simulink model "c960x4096_x14_7_r2013b_frb"  (R2013b)
settings: Solver=ode45  StartTime=0.0  StopTime=40960  RelTol=1e-3
undefined symbols (not defined in the file): sfp
libraries: xbsIndex_r4 x14620, casper_library_misc x61, dspsigops x32, casper_library_multipliers x24, simulink x18, xps_library x18
(part 9 of 79)

== system c960x4096_x14_7_r2013b_frb/cross_corr/cross_multiplier ==
  sync_in : Inport
  din0 : Inport  Port=2
  din1 : Inport  Port=3
  c_to_ri0_{0..7} (8 alike) : casper_library_misc/c_to_ri  n_bits=bit_width_in  bin_pt=binary_point_in
  c_to_ri1_{0..7} (8 alike) : casper_library_misc/c_to_ri  n_bits=bit_width_in  bin_pt=binary_point_in
  cmult0_0_{0..7} (8 alike) : casper_library_multipliers/cmult_4bit_hdl*  mult_latency=mult_latency  add_latency=add_latency
  cmult0_1_{0..7} (8 alike) : casper_library_multipliers/cmult_4bit_hdl*  mult_latency=mult_latency  add_latency=add_latency
  cmult1_0_{0..7} (8 alike) : casper_library_multipliers/cmult_4bit_hdl*  mult_latency=mult_latency  add_latency=add_latency
  cvrt0_0_0_imag : Subsystem  AncestorBlock=casper_library_misc/convert_of  mask(convert_of){bit_width_i=37, binary_point_i=34, bit_width_o=37, binary_point_o=34, latency=0, overflow=Wrap, quantization=Truncate}
      mask prompts: bit_width_i "Bit Width In"; binary_point_i "Binary Point In"; bit_width_o "Bit Width Out"; binary_point_o "Binary Point Out"; overflow "Overflow Behaviour"; quantization "Quantization Behaviour"
      mask help:
      | Converts from one 2's complement bit-width
      | and/or binary point position to another.
      | Includes underflow/overflow indicator.
      mask init:
      | convert_of_init(gcb, ...
      |     'bit_width_i', bit_width_i, ...
      |     'binary_point_i', binary_point_i, ...
      |     'bit_width_o', bit_width_o, ...
      |     'binary_point_o', binary_point_o, ...
      |     'latency', latency, ...
      |     'overflow', overflow, ...
      |     'quantization', quantization);
      settings: AttributesFormatString=[37,34]->[37,34]
      mask TypeOptions overflow: Wrap | Saturate | Error
      mask TypeOptions quantization: Truncate | Round  (unbiased: +/- Inf) | Round  (unbiased: even values)
  cvrt0_0_0_real : Subsystem  AncestorBlock=casper_library_misc/convert_of  mask(convert_of){bit_width_i=37, binary_point_i=34, bit_width_o=37, binary_point_o=34, latency=0, overflow=Wrap, quantization=Truncate}
      mask prompts: bit_width_i "Bit Width In"; binary_point_i "Binary Point In"; bit_width_o "Bit Width Out"; binary_point_o "Binary Point Out"; overflow "Overflow Behaviour"; quantization "Quantization Behaviour"
      mask help:
      | Converts from one 2's complement bit-width
      | and/or binary point position to another.
      | Includes underflow/overflow indicator.
      mask init: same as c960x4096_x14_7_r2013b_frb/cross_corr/cross_multiplier/cvrt0_0_0_imag
      settings: AttributesFormatString=[37,34]->[37,34]
      mask TypeOptions overflow: Wrap | Saturate | Error
      mask TypeOptions quantization: Truncate | Round  (unbiased: +/- Inf) | Round  (unbiased: even values)
  cvrt0_0_1_imag : Subsystem  AncestorBlock=casper_library_misc/convert_of  mask(convert_of){bit_width_i=37, binary_point_i=34, bit_width_o=37, binary_point_o=34, latency=0, overflow=Wrap, quantization=Truncate}
      mask prompts: bit_width_i "Bit Width In"; binary_point_i "Binary Point In"; bit_width_o "Bit Width Out"; binary_point_o "Binary Point Out"; overflow "Overflow Behaviour"; quantization "Quantization Behaviour"
      mask help:
      | Converts from one 2's complement bit-width
      | and/or binary point position to another.
      | Includes underflow/overflow indicator.
      mask init: same as c960x4096_x14_7_r2013b_frb/cross_corr/cross_multiplier/cvrt0_0_0_imag
      settings: AttributesFormatString=[37,34]->[37,34]
      mask TypeOptions overflow: Wrap | Saturate | Error
      mask TypeOptions quantization: Truncate | Round  (unbiased: +/- Inf) | Round  (unbiased: even values)
  cvrt0_0_1_real : Subsystem  AncestorBlock=casper_library_misc/convert_of  mask(convert_of){bit_width_i=37, binary_point_i=34, bit_width_o=37, binary_point_o=34, latency=0, overflow=Wrap, quantization=Truncate}
      mask prompts: bit_width_i "Bit Width In"; binary_point_i "Binary Point In"; bit_width_o "Bit Width Out"; binary_point_o "Binary Point Out"; overflow "Overflow Behaviour"; quantization "Quantization Behaviour"
      mask help:
      | Converts from one 2's complement bit-width
      | and/or binary point position to another.
      | Includes underflow/overflow indicator.
      mask init: same as c960x4096_x14_7_r2013b_frb/cross_corr/cross_multiplier/cvrt0_0_0_imag
      settings: AttributesFormatString=[37,34]->[37,34]
      mask TypeOptions overflow: Wrap | Saturate | Error
      mask TypeOptions quantization: Truncate | Round  (unbiased: +/- Inf) | Round  (unbiased: even values)
  cvrt0_0_2_imag : Subsystem  AncestorBlock=casper_library_misc/convert_of  mask(convert_of){bit_width_i=37, binary_point_i=34, bit_width_o=37, binary_point_o=34, latency=0, overflow=Wrap, quantization=Truncate}
      mask prompts: bit_width_i "Bit Width In"; binary_point_i "Binary Point In"; bit_width_o "Bit Width Out"; binary_point_o "Binary Point Out"; overflow "Overflow Behaviour"; quantization "Quantization Behaviour"
      mask help:
      | Converts from one 2's complement bit-width
      | and/or binary point position to another.
      | Includes underflow/overflow indicator.
      mask init: same as c960x4096_x14_7_r2013b_frb/cross_corr/cross_multiplier/cvrt0_0_0_imag
      settings: AttributesFormatString=[37,34]->[37,34]
      mask TypeOptions overflow: Wrap | Saturate | Error
      mask TypeOptions quantization: Truncate | Round  (unbiased: +/- Inf) | Round  (unbiased: even values)
  cvrt0_0_2_real : Subsystem  AncestorBlock=casper_library_misc/convert_of  mask(convert_of){bit_width_i=37, binary_point_i=34, bit_width_o=37, binary_point_o=34, latency=0, overflow=Wrap, quantization=Truncate}
      mask prompts: bit_width_i "Bit Width In"; binary_point_i "Binary Point In"; bit_width_o "Bit Width Out"; binary_point_o "Binary Point Out"; overflow "Overflow Behaviour"; quantization "Quantization Behaviour"
      mask help:
      | Converts from one 2's complement bit-width
      | and/or binary point position to another.
      | Includes underflow/overflow indicator.
      mask init: same as c960x4096_x14_7_r2013b_frb/cross_corr/cross_multiplier/cvrt0_0_0_imag
      settings: AttributesFormatString=[37,34]->[37,34]
      mask TypeOptions overflow: Wrap | Saturate | Error
      mask TypeOptions quantization: Truncate | Round  (unbiased: +/- Inf) | Round  (unbiased: even values)
  cvrt0_0_3_imag : Subsystem  AncestorBlock=casper_library_misc/convert_of  mask(convert_of){bit_width_i=37, binary_point_i=34, bit_width_o=37, binary_point_o=34, latency=0, overflow=Wrap, quantization=Truncate}
      mask prompts: bit_width_i "Bit Width In"; binary_point_i "Binary Point In"; bit_width_o "Bit Width Out"; binary_point_o "Binary Point Out"; overflow "Overflow Behaviour"; quantization "Quantization Behaviour"
      mask help:
      | Converts from one 2's complement bit-width
      | and/or binary point position to another.
      | Includes underflow/overflow indicator.
      mask init: same as c960x4096_x14_7_r2013b_frb/cross_corr/cross_multiplier/cvrt0_0_0_imag
      settings: AttributesFormatString=[37,34]->[37,34]
      mask TypeOptions overflow: Wrap | Saturate | Error
      mask TypeOptions quantization: Truncate | Round  (unbiased: +/- Inf) | Round  (unbiased: even values)
  cvrt0_0_3_real : Subsystem  AncestorBlock=casper_library_misc/convert_of  mask(convert_of){bit_width_i=37, binary_point_i=34, bit_width_o=37, binary_point_o=34, latency=0, overflow=Wrap, quantization=Truncate}
      mask prompts: bit_width_i "Bit Width In"; binary_point_i "Binary Point In"; bit_width_o "Bit Width Out"; binary_point_o "Binary Point Out"; overflow "Overflow Behaviour"; quantization "Quantization Behaviour"
      mask help:
      | Converts from one 2's complement bit-width
      | and/or binary point position to another.
      | Includes underflow/overflow indicator.
      mask init: same as c960x4096_x14_7_r2013b_frb/cross_corr/cross_multiplier/cvrt0_0_0_imag
      settings: AttributesFormatString=[37,34]->[37,34]
      mask TypeOptions overflow: Wrap | Saturate | Error
      mask TypeOptions quantization: Truncate | Round  (unbiased: +/- Inf) | Round  (unbiased: even values)
  cvrt0_0_4_imag : Subsystem  AncestorBlock=casper_library_misc/convert_of  mask(convert_of){bit_width_i=37, binary_point_i=34, bit_width_o=37, binary_point_o=34, latency=0, overflow=Wrap, quantization=Truncate}
      mask prompts: bit_width_i "Bit Width In"; binary_point_i "Binary Point In"; bit_width_o "Bit Width Out"; binary_point_o "Binary Point Out"; overflow "Overflow Behaviour"; quantization "Quantization Behaviour"
      mask help:
      | Converts from one 2's complement bit-width
      | and/or binary point position to another.
      | Includes underflow/overflow indicator.
      mask init: same as c960x4096_x14_7_r2013b_frb/cross_corr/cross_multiplier/cvrt0_0_0_imag
      settings: AttributesFormatString=[37,34]->[37,34]
      mask TypeOptions overflow: Wrap | Saturate | Error
      mask TypeOptions quantization: Truncate | Round  (unbiased: +/- Inf) | Round  (unbiased: even values)
  cvrt0_0_4_real : Subsystem  AncestorBlock=casper_library_misc/convert_of  mask(convert_of){bit_width_i=37, binary_point_i=34, bit_width_o=37, binary_point_o=34, latency=0, overflow=Wrap, quantization=Truncate}
      mask prompts: bit_width_i "Bit Width In"; binary_point_i "Binary Point In"; bit_width_o "Bit Width Out"; binary_point_o "Binary Point Out"; overflow "Overflow Behaviour"; quantization "Quantization Behaviour"
      mask help:
      | Converts from one 2's complement bit-width
      | and/or binary point position to another.
      | Includes underflow/overflow indicator.
      mask init: same as c960x4096_x14_7_r2013b_frb/cross_corr/cross_multiplier/cvrt0_0_0_imag
      settings: AttributesFormatString=[37,34]->[37,34]
      mask TypeOptions overflow: Wrap | Saturate | Error
      mask TypeOptions quantization: Truncate | Round  (unbiased: +/- Inf) | Round  (unbiased: even values)
  cvrt0_0_5_imag : Subsystem  AncestorBlock=casper_library_misc/convert_of  mask(convert_of){bit_width_i=37, binary_point_i=34, bit_width_o=37, binary_point_o=34, latency=0, overflow=Wrap, quantization=Truncate}
      mask prompts: bit_width_i "Bit Width In"; binary_point_i "Binary Point In"; bit_width_o "Bit Width Out"; binary_point_o "Binary Point Out"; overflow "Overflow Behaviour"; quantization "Quantization Behaviour"
      mask help:
      | Converts from one 2's complement bit-width
      | and/or binary point position to another.
      | Includes underflow/overflow indicator.
      mask init: same as c960x4096_x14_7_r2013b_frb/cross_corr/cross_multiplier/cvrt0_0_0_imag
      settings: AttributesFormatString=[37,34]->[37,34]
      mask TypeOptions overflow: Wrap | Saturate | Error
      mask TypeOptions quantization: Truncate | Round  (unbiased: +/- Inf) | Round  (unbiased: even values)
  cvrt0_0_5_real : Subsystem  AncestorBlock=casper_library_misc/convert_of  mask(convert_of){bit_width_i=37, binary_point_i=34, bit_width_o=37, binary_point_o=34, latency=0, overflow=Wrap, quantization=Truncate}
      mask prompts: bit_width_i "Bit Width In"; binary_point_i "Binary Point In"; bit_width_o "Bit Width Out"; binary_point_o "Binary Point Out"; overflow "Overflow Behaviour"; quantization "Quantization Behaviour"
      mask help:
      | Converts from one 2's complement bit-width
      | and/or binary point position to another.
      | Includes underflow/overflow indicator.
      mask init: same as c960x4096_x14_7_r2013b_frb/cross_corr/cross_multiplier/cvrt0_0_0_imag
      settings: AttributesFormatString=[37,34]->[37,34]
      mask TypeOptions overflow: Wrap | Saturate | Error
      mask TypeOptions quantization: Truncate | Round  (unbiased: +/- Inf) | Round  (unbiased: even values)
  cvrt0_0_6_imag : Subsystem  AncestorBlock=casper_library_misc/convert_of  mask(convert_of){bit_width_i=37, binary_point_i=34, bit_width_o=37, binary_point_o=34, latency=0, overflow=Wrap, quantization=Truncate}
      mask prompts: bit_width_i "Bit Width In"; binary_point_i "Binary Point In"; bit_width_o "Bit Width Out"; binary_point_o "Binary Point Out"; overflow "Overflow Behaviour"; quantization "Quantization Behaviour"
      mask help:
      | Converts from one 2's complement bit-width
      | and/or binary point position to another.
      | Includes underflow/overflow indicator.
      mask init: same as c960x4096_x14_7_r2013b_frb/cross_corr/cross_multiplier/cvrt0_0_0_imag
      settings: AttributesFormatString=[37,34]->[37,34]
      mask TypeOptions overflow: Wrap | Saturate | Error
      mask TypeOptions quantization: Truncate | Round  (unbiased: +/- Inf) | Round  (unbiased: even values)
  cvrt0_0_6_real : Subsystem  AncestorBlock=casper_library_misc/convert_of  mask(convert_of){bit_width_i=37, binary_point_i=34, bit_width_o=37, binary_point_o=34, latency=0, overflow=Wrap, quantization=Truncate}
      mask prompts: bit_width_i "Bit Width In"; binary_point_i "Binary Point In"; bit_width_o "Bit Width Out"; binary_point_o "Binary Point Out"; overflow "Overflow Behaviour"; quantization "Quantization Behaviour"
      mask help:
      | Converts from one 2's complement bit-width
      | and/or binary point position to another.
      | Includes underflow/overflow indicator.
      mask init: same as c960x4096_x14_7_r2013b_frb/cross_corr/cross_multiplier/cvrt0_0_0_imag
      settings: AttributesFormatString=[37,34]->[37,34]
      mask TypeOptions overflow: Wrap | Saturate | Error
      mask TypeOptions quantization: Truncate | Round  (unbiased: +/- Inf) | Round  (unbiased: even values)
  cvrt0_0_7_imag : Subsystem  AncestorBlock=casper_library_misc/convert_of  mask(convert_of){bit_width_i=37, binary_point_i=34, bit_width_o=37, binary_point_o=34, latency=0, overflow=Wrap, quantization=Truncate}
      mask prompts: bit_width_i "Bit Width In"; binary_point_i "Binary Point In"; bit_width_o "Bit Width Out"; binary_point_o "Binary Point Out"; overflow "Overflow Behaviour"; quantization "Quantization Behaviour"
      mask help:
      | Converts from one 2's complement bit-width
      | and/or binary point position to another.
      | Includes underflow/overflow indicator.
      mask init: same as c960x4096_x14_7_r2013b_frb/cross_corr/cross_multiplier/cvrt0_0_0_imag
      settings: AttributesFormatString=[37,34]->[37,34]
      mask TypeOptions overflow: Wrap | Saturate | Error
      mask TypeOptions quantization: Truncate | Round  (unbiased: +/- Inf) | Round  (unbiased: even values)
  cvrt0_0_7_real : Subsystem  AncestorBlock=casper_library_misc/convert_of  mask(convert_of){bit_width_i=37, binary_point_i=34, bit_width_o=37, binary_point_o=34, latency=0, overflow=Wrap, quantization=Truncate}
      mask prompts: bit_width_i "Bit Width In"; binary_point_i "Binary Point In"; bit_width_o "Bit Width Out"; binary_point_o "Binary Point Out"; overflow "Overflow Behaviour"; quantization "Quantization Behaviour"
      mask help:
      | Converts from one 2's complement bit-width
      | and/or binary point position to another.
      | Includes underflow/overflow indicator.
      mask init: same as c960x4096_x14_7_r2013b_frb/cross_corr/cross_multiplier/cvrt0_0_0_imag
      settings: AttributesFormatString=[37,34]->[37,34]
      mask TypeOptions overflow: Wrap | Saturate | Error
      mask TypeOptions quantization: Truncate | Round  (unbiased: +/- Inf) | Round  (unbiased: even values)
  cvrt0_1_0_imag : Subsystem  AncestorBlock=casper_library_misc/convert_of  mask(convert_of){bit_width_i=37, binary_point_i=34, bit_width_o=37, binary_point_o=34, latency=0, overflow=Wrap, quantization=Truncate}
      mask prompts: bit_width_i "Bit Width In"; binary_point_i "Binary Point In"; bit_width_o "Bit Width Out"; binary_point_o "Binary Point Out"; overflow "Overflow Behaviour"; quantization "Quantization Behaviour"
      mask help:
      | Converts from one 2's complement bit-width
      | and/or binary point position to another.
      | Includes underflow/overflow indicator.
      mask init: same as c960x4096_x14_7_r2013b_frb/cross_corr/cross_multiplier/cvrt0_0_0_imag
      settings: AttributesFormatString=[37,34]->[37,34]
      mask TypeOptions overflow: Wrap | Saturate | Error
      mask TypeOptions quantization: Truncate | Round  (unbiased: +/- Inf) | Round  (unbiased: even values)
  cvrt0_1_0_real : Subsystem  AncestorBlock=casper_library_misc/convert_of  mask(convert_of){bit_width_i=37, binary_point_i=34, bit_width_o=37, binary_point_o=34, latency=0, overflow=Wrap, quantization=Truncate}
      mask prompts: bit_width_i "Bit Width In"; binary_point_i "Binary Point In"; bit_width_o "Bit Width Out"; binary_point_o "Binary Point Out"; overflow "Overflow Behaviour"; quantization "Quantization Behaviour"
      mask help:
      | Converts from one 2's complement bit-width
      | and/or binary point position to another.
      | Includes underflow/overflow indicator.
      mask init: same as c960x4096_x14_7_r2013b_frb/cross_corr/cross_multiplier/cvrt0_0_0_imag
      settings: AttributesFormatString=[37,34]->[37,34]
      mask TypeOptions overflow: Wrap | Saturate | Error
      mask TypeOptions quantization: Truncate | Round  (unbiased: +/- Inf) | Round  (unbiased: even values)
  cvrt0_1_1_imag : Subsystem  AncestorBlock=casper_library_misc/convert_of  mask(convert_of){bit_width_i=37, binary_point_i=34, bit_width_o=37, binary_point_o=34, latency=0, overflow=Wrap, quantization=Truncate}
      mask prompts: bit_width_i "Bit Width In"; binary_point_i "Binary Point In"; bit_width_o "Bit Width Out"; binary_point_o "Binary Point Out"; overflow "Overflow Behaviour"; quantization "Quantization Behaviour"
      mask help:
      | Converts from one 2's complement bit-width
      | and/or binary point position to another.
      | Includes underflow/overflow indicator.
      mask init: same as c960x4096_x14_7_r2013b_frb/cross_corr/cross_multiplier/cvrt0_0_0_imag
      settings: AttributesFormatString=[37,34]->[37,34]
      mask TypeOptions overflow: Wrap | Saturate | Error
      mask TypeOptions quantization: Truncate | Round  (unbiased: +/- Inf) | Round  (unbiased: even values)
  cvrt0_1_1_real : Subsystem  AncestorBlock=casper_library_misc/convert_of  mask(convert_of){bit_width_i=37, binary_point_i=34, bit_width_o=37, binary_point_o=34, latency=0, overflow=Wrap, quantization=Truncate}
      mask prompts: bit_width_i "Bit Width In"; binary_point_i "Binary Point In"; bit_width_o "Bit Width Out"; binary_point_o "Binary Point Out"; overflow "Overflow Behaviour"; quantization "Quantization Behaviour"
      mask help:
      | Converts from one 2's complement bit-width
      | and/or binary point position to another.
      | Includes underflow/overflow indicator.
      mask init: same as c960x4096_x14_7_r2013b_frb/cross_corr/cross_multiplier/cvrt0_0_0_imag
      settings: AttributesFormatString=[37,34]->[37,34]
      mask TypeOptions overflow: Wrap | Saturate | Error
      mask TypeOptions quantization: Truncate | Round  (unbiased: +/- Inf) | Round  (unbiased: even values)
  cvrt0_1_2_imag : Subsystem  AncestorBlock=casper_library_misc/convert_of  mask(convert_of){bit_width_i=37, binary_point_i=34, bit_width_o=37, binary_point_o=34, latency=0, overflow=Wrap, quantization=Truncate}
      mask prompts: bit_width_i "Bit Width In"; binary_point_i "Binary Point In"; bit_width_o "Bit Width Out"; binary_point_o "Binary Point Out"; overflow "Overflow Behaviour"; quantization "Quantization Behaviour"
      mask help:
      | Converts from one 2's complement bit-width
      | and/or binary point position to another.
      | Includes underflow/overflow indicator.
      mask init: same as c960x4096_x14_7_r2013b_frb/cross_corr/cross_multiplier/cvrt0_0_0_imag
      settings: AttributesFormatString=[37,34]->[37,34]
      mask TypeOptions overflow: Wrap | Saturate | Error
      mask TypeOptions quantization: Truncate | Round  (unbiased: +/- Inf) | Round  (unbiased: even values)
  cvrt0_1_2_real : Subsystem  AncestorBlock=casper_library_misc/convert_of  mask(convert_of){bit_width_i=37, binary_point_i=34, bit_width_o=37, binary_point_o=34, latency=0, overflow=Wrap, quantization=Truncate}
      mask prompts: bit_width_i "Bit Width In"; binary_point_i "Binary Point In"; bit_width_o "Bit Width Out"; binary_point_o "Binary Point Out"; overflow "Overflow Behaviour"; quantization "Quantization Behaviour"
      mask help:
      | Converts from one 2's complement bit-width
      | and/or binary point position to another.
      | Includes underflow/overflow indicator.
      mask init: same as c960x4096_x14_7_r2013b_frb/cross_corr/cross_multiplier/cvrt0_0_0_imag
      settings: AttributesFormatString=[37,34]->[37,34]
      mask TypeOptions overflow: Wrap | Saturate | Error
      mask TypeOptions quantization: Truncate | Round  (unbiased: +/- Inf) | Round  (unbiased: even values)
  cvrt0_1_3_imag : Subsystem  AncestorBlock=casper_library_misc/convert_of  mask(convert_of){bit_width_i=37, binary_point_i=34, bit_width_o=37, binary_point_o=34, latency=0, overflow=Wrap, quantization=Truncate}
      mask prompts: bit_width_i "Bit Width In"; binary_point_i "Binary Point In"; bit_width_o "Bit Width Out"; binary_point_o "Binary Point Out"; overflow "Overflow Behaviour"; quantization "Quantization Behaviour"
      mask help:
      | Converts from one 2's complement bit-width
      | and/or binary point position to another.
      | Includes underflow/overflow indicator.
      mask init: same as c960x4096_x14_7_r2013b_frb/cross_corr/cross_multiplier/cvrt0_0_0_imag
      settings: AttributesFormatString=[37,34]->[37,34]
      mask TypeOptions overflow: Wrap | Saturate | Error
      mask TypeOptions quantization: Truncate | Round  (unbiased: +/- Inf) | Round  (unbiased: even values)
  cvrt0_1_3_real : Subsystem  AncestorBlock=casper_library_misc/convert_of  mask(convert_of){bit_width_i=37, binary_point_i=34, bit_width_o=37, binary_point_o=34, latency=0, overflow=Wrap, quantization=Truncate}
      mask prompts: bit_width_i "Bit Width In"; binary_point_i "Binary Point In"; bit_width_o "Bit Width Out"; binary_point_o "Binary Point Out"; overflow "Overflow Behaviour"; quantization "Quantization Behaviour"
      mask help:
      | Converts from one 2's complement bit-width
      | and/or binary point position to another.
      | Includes underflow/overflow indicator.
      mask init: same as c960x4096_x14_7_r2013b_frb/cross_corr/cross_multiplier/cvrt0_0_0_imag
      settings: AttributesFormatString=[37,34]->[37,34]
      mask TypeOptions overflow: Wrap | Saturate | Error
      mask TypeOptions quantization: Truncate | Round  (unbiased: +/- Inf) | Round  (unbiased: even values)
  cvrt0_1_4_imag : Subsystem  AncestorBlock=casper_library_misc/convert_of  mask(convert_of){bit_width_i=37, binary_point_i=34, bit_width_o=37, binary_point_o=34, latency=0, overflow=Wrap, quantization=Truncate}
      mask prompts: bit_width_i "Bit Width In"; binary_point_i "Binary Point In"; bit_width_o "Bit Width Out"; binary_point_o "Binary Point Out"; overflow "Overflow Behaviour"; quantization "Quantization Behaviour"
      mask help:
      | Converts from one 2's complement bit-width
      | and/or binary point position to another.
      | Includes underflow/overflow indicator.
      mask init: same as c960x4096_x14_7_r2013b_frb/cross_corr/cross_multiplier/cvrt0_0_0_imag
      settings: AttributesFormatString=[37,34]->[37,34]
      mask TypeOptions overflow: Wrap | Saturate | Error
      mask TypeOptions quantization: Truncate | Round  (unbiased: +/- Inf) | Round  (unbiased: even values)
  cvrt0_1_4_real : Subsystem  AncestorBlock=casper_library_misc/convert_of  mask(convert_of){bit_width_i=37, binary_point_i=34, bit_width_o=37, binary_point_o=34, latency=0, overflow=Wrap, quantization=Truncate}
      mask prompts: bit_width_i "Bit Width In"; binary_point_i "Binary Point In"; bit_width_o "Bit Width Out"; binary_point_o "Binary Point Out"; overflow "Overflow Behaviour"; quantization "Quantization Behaviour"
      mask help:
      | Converts from one 2's complement bit-width
      | and/or binary point position to another.
      | Includes underflow/overflow indicator.
      mask init: same as c960x4096_x14_7_r2013b_frb/cross_corr/cross_multiplier/cvrt0_0_0_imag
      settings: AttributesFormatString=[37,34]->[37,34]
      mask TypeOptions overflow: Wrap | Saturate | Error
      mask TypeOptions quantization: Truncate | Round  (unbiased: +/- Inf) | Round  (unbiased: even values)
  cvrt0_1_5_imag : Subsystem  AncestorBlock=casper_library_misc/convert_of  mask(convert_of){bit_width_i=37, binary_point_i=34, bit_width_o=37, binary_point_o=34, latency=0, overflow=Wrap, quantization=Truncate}
      mask prompts: bit_width_i "Bit Width In"; binary_point_i "Binary Point In"; bit_width_o "Bit Width Out"; binary_point_o "Binary Point Out"; overflow "Overflow Behaviour"; quantization "Quantization Behaviour"
      mask help:
      | Converts from one 2's complement bit-width
      | and/or binary point position to another.
      | Includes underflow/overflow indicator.
      mask init: same as c960x4096_x14_7_r2013b_frb/cross_corr/cross_multiplier/cvrt0_0_0_imag
      settings: AttributesFormatString=[37,34]->[37,34]
      mask TypeOptions overflow: Wrap | Saturate | Error
      mask TypeOptions quantization: Truncate | Round  (unbiased: +/- Inf) | Round  (unbiased: even values)
  cvrt0_1_5_real : Subsystem  AncestorBlock=casper_library_misc/convert_of  mask(convert_of){bit_width_i=37, binary_point_i=34, bit_width_o=37, binary_point_o=34, latency=0, overflow=Wrap, quantization=Truncate}
      mask prompts: bit_width_i "Bit Width In"; binary_point_i "Binary Point In"; bit_width_o "Bit Width Out"; binary_point_o "Binary Point Out"; overflow "Overflow Behaviour"; quantization "Quantization Behaviour"
      mask help:
      | Converts from one 2's complement bit-width
      | and/or binary point position to another.
      | Includes underflow/overflow indicator.
      mask init: same as c960x4096_x14_7_r2013b_frb/cross_corr/cross_multiplier/cvrt0_0_0_imag
      settings: AttributesFormatString=[37,34]->[37,34]
      mask TypeOptions overflow: Wrap | Saturate | Error
      mask TypeOptions quantization: Truncate | Round  (unbiased: +/- Inf) | Round  (unbiased: even values)
  cvrt0_1_6_imag : Subsystem  AncestorBlock=casper_library_misc/convert_of  mask(convert_of){bit_width_i=37, binary_point_i=34, bit_width_o=37, binary_point_o=34, latency=0, overflow=Wrap, quantization=Truncate}
      mask prompts: bit_width_i "Bit Width In"; binary_point_i "Binary Point In"; bit_width_o "Bit Width Out"; binary_point_o "Binary Point Out"; overflow "Overflow Behaviour"; quantization "Quantization Behaviour"
      mask help:
      | Converts from one 2's complement bit-width
      | and/or binary point position to another.
      | Includes underflow/overflow indicator.
      mask init: same as c960x4096_x14_7_r2013b_frb/cross_corr/cross_multiplier/cvrt0_0_0_imag
      settings: AttributesFormatString=[37,34]->[37,34]
      mask TypeOptions overflow: Wrap | Saturate | Error
      mask TypeOptions quantization: Truncate | Round  (unbiased: +/- Inf) | Round  (unbiased: even values)
  cvrt0_1_6_real : Subsystem  AncestorBlock=casper_library_misc/convert_of  mask(convert_of){bit_width_i=37, binary_point_i=34, bit_width_o=37, binary_point_o=34, latency=0, overflow=Wrap, quantization=Truncate}
      mask prompts: bit_width_i "Bit Width In"; binary_point_i "Binary Point In"; bit_width_o "Bit Width Out"; binary_point_o "Binary Point Out"; overflow "Overflow Behaviour"; quantization "Quantization Behaviour"
      mask help:
      | Converts from one 2's complement bit-width
      | and/or binary point position to another.
      | Includes underflow/overflow indicator.
      mask init: same as c960x4096_x14_7_r2013b_frb/cross_corr/cross_multiplier/cvrt0_0_0_imag
      settings: AttributesFormatString=[37,34]->[37,34]
      mask TypeOptions overflow: Wrap | Saturate | Error
      mask TypeOptions quantization: Truncate | Round  (unbiased: +/- Inf) | Round  (unbiased: even values)
  cvrt0_1_7_imag : Subsystem  AncestorBlock=casper_library_misc/convert_of  mask(convert_of){bit_width_i=37, binary_point_i=34, bit_width_o=37, binary_point_o=34, latency=0, overflow=Wrap, quantization=Truncate}
      mask prompts: bit_width_i "Bit Width In"; binary_point_i "Binary Point In"; bit_width_o "Bit Width Out"; binary_point_o "Binary Point Out"; overflow "Overflow Behaviour"; quantization "Quantization Behaviour"
      mask help:
      | Converts from one 2's complement bit-width
      | and/or binary point position to another.
      | Includes underflow/overflow indicator.
      mask init: same as c960x4096_x14_7_r2013b_frb/cross_corr/cross_multiplier/cvrt0_0_0_imag
      settings: AttributesFormatString=[37,34]->[37,34]
      mask TypeOptions overflow: Wrap | Saturate | Error
      mask TypeOptions quantization: Truncate | Round  (unbiased: +/- Inf) | Round  (unbiased: even values)
  cvrt0_1_7_real : Subsystem  AncestorBlock=casper_library_misc/convert_of  mask(convert_of){bit_width_i=37, binary_point_i=34, bit_width_o=37, binary_point_o=34, latency=0, overflow=Wrap, quantization=Truncate}
      mask prompts: bit_width_i "Bit Width In"; binary_point_i "Binary Point In"; bit_width_o "Bit Width Out"; binary_point_o "Binary Point Out"; overflow "Overflow Behaviour"; quantization "Quantization Behaviour"
      mask help:
      | Converts from one 2's complement bit-width
      | and/or binary point position to another.
      | Includes underflow/overflow indicator.
      mask init: same as c960x4096_x14_7_r2013b_frb/cross_corr/cross_multiplier/cvrt0_0_0_imag
      settings: AttributesFormatString=[37,34]->[37,34]
      mask TypeOptions overflow: Wrap | Saturate | Error
      mask TypeOptions quantization: Truncate | Round  (unbiased: +/- Inf) | Round  (unbiased: even values)
  cvrt1_0_0_imag : Subsystem  AncestorBlock=casper_library_misc/convert_of  mask(convert_of){bit_width_i=37, binary_point_i=34, bit_width_o=37, binary_point_o=34, latency=0, overflow=Wrap, quantization=Truncate}
      mask prompts: bit_width_i "Bit Width In"; binary_point_i "Binary Point In"; bit_width_o "Bit Width Out"; binary_point_o "Binary Point Out"; overflow "Overflow Behaviour"; quantization "Quantization Behaviour"
      mask help:
      | Converts from one 2's complement bit-width
      | and/or binary point position to another.
      | Includes underflow/overflow indicator.
      mask init: same as c960x4096_x14_7_r2013b_frb/cross_corr/cross_multiplier/cvrt0_0_0_imag
      settings: AttributesFormatString=[37,34]->[37,34]
      mask TypeOptions overflow: Wrap | Saturate | Error
      mask TypeOptions quantization: Truncate | Round  (unbiased: +/- Inf) | Round  (unbiased: even values)
  cvrt1_0_0_real : Subsystem  AncestorBlock=casper_library_misc/convert_of  mask(convert_of){bit_width_i=37, binary_point_i=34, bit_width_o=37, binary_point_o=34, latency=0, overflow=Wrap, quantization=Truncate}
      mask prompts: bit_width_i "Bit Width In"; binary_point_i "Binary Point In"; bit_width_o "Bit Width Out"; binary_point_o "Binary Point Out"; overflow "Overflow Behaviour"; quantization "Quantization Behaviour"
      mask help:
      | Converts from one 2's complement bit-width
      | and/or binary point position to another.
      | Includes underflow/overflow indicator.
      mask init: same as c960x4096_x14_7_r2013b_frb/cross_corr/cross_multiplier/cvrt0_0_0_imag
      settings: AttributesFormatString=[37,34]->[37,34]
      mask TypeOptions overflow: Wrap | Saturate | Error
      mask TypeOptions quantization: Truncate | Round  (unbiased: +/- Inf) | Round  (unbiased: even values)
  cvrt1_0_1_imag : Subsystem  AncestorBlock=casper_library_misc/convert_of  mask(convert_of){bit_width_i=37, binary_point_i=34, bit_width_o=37, binary_point_o=34, latency=0, overflow=Wrap, quantization=Truncate}
      mask prompts: bit_width_i "Bit Width In"; binary_point_i "Binary Point In"; bit_width_o "Bit Width Out"; binary_point_o "Binary Point Out"; overflow "Overflow Behaviour"; quantization "Quantization Behaviour"
      mask help:
      | Converts from one 2's complement bit-width
      | and/or binary point position to another.
      | Includes underflow/overflow indicator.
      mask init: same as c960x4096_x14_7_r2013b_frb/cross_corr/cross_multiplier/cvrt0_0_0_imag
      settings: AttributesFormatString=[37,34]->[37,34]
      mask TypeOptions overflow: Wrap | Saturate | Error
      mask TypeOptions quantization: Truncate | Round  (unbiased: +/- Inf) | Round  (unbiased: even values)
  cvrt1_0_1_real : Subsystem  AncestorBlock=casper_library_misc/convert_of  mask(convert_of){bit_width_i=37, binary_point_i=34, bit_width_o=37, binary_point_o=34, latency=0, overflow=Wrap, quantization=Truncate}
      mask prompts: bit_width_i "Bit Width In"; binary_point_i "Binary Point In"; bit_width_o "Bit Width Out"; binary_point_o "Binary Point Out"; overflow "Overflow Behaviour"; quantization "Quantization Behaviour"
      mask help:
      | Converts from one 2's complement bit-width
      | and/or binary point position to another.
      | Includes underflow/overflow indicator.
      mask init: same as c960x4096_x14_7_r2013b_frb/cross_corr/cross_multiplier/cvrt0_0_0_imag
      settings: AttributesFormatString=[37,34]->[37,34]
      mask TypeOptions overflow: Wrap | Saturate | Error
      mask TypeOptions quantization: Truncate | Round  (unbiased: +/- Inf) | Round  (unbiased: even values)
  cvrt1_0_2_imag : Subsystem  AncestorBlock=casper_library_misc/convert_of  mask(convert_of){bit_width_i=37, binary_point_i=34, bit_width_o=37, binary_point_o=34, latency=0, overflow=Wrap, quantization=Truncate}
      mask prompts: bit_width_i "Bit Width In"; binary_point_i "Binary Point In"; bit_width_o "Bit Width Out"; binary_point_o "Binary Point Out"; overflow "Overflow Behaviour"; quantization "Quantization Behaviour"
      mask help:
      | Converts from one 2's complement bit-width
      | and/or binary point position to another.
      | Includes underflow/overflow indicator.
      mask init: same as c960x4096_x14_7_r2013b_frb/cross_corr/cross_multiplier/cvrt0_0_0_imag
      settings: AttributesFormatString=[37,34]->[37,34]
      mask TypeOptions overflow: Wrap | Saturate | Error
      mask TypeOptions quantization: Truncate | Round  (unbiased: +/- Inf) | Round  (unbiased: even values)
  cvrt1_0_2_real : Subsystem  AncestorBlock=casper_library_misc/convert_of  mask(convert_of){bit_width_i=37, binary_point_i=34, bit_width_o=37, binary_point_o=34, latency=0, overflow=Wrap, quantization=Truncate}
      mask prompts: bit_width_i "Bit Width In"; binary_point_i "Binary Point In"; bit_width_o "Bit Width Out"; binary_point_o "Binary Point Out"; overflow "Overflow Behaviour"; quantization "Quantization Behaviour"
      mask help:
      | Converts from one 2's complement bit-width
      | and/or binary point position to another.
      | Includes underflow/overflow indicator.
      mask init: same as c960x4096_x14_7_r2013b_frb/cross_corr/cross_multiplier/cvrt0_0_0_imag
      settings: AttributesFormatString=[37,34]->[37,34]
      mask TypeOptions overflow: Wrap | Saturate | Error
      mask TypeOptions quantization: Truncate | Round  (unbiased: +/- Inf) | Round  (unbiased: even values)
  cvrt1_0_3_imag : Subsystem  AncestorBlock=casper_library_misc/convert_of  mask(convert_of){bit_width_i=37, binary_point_i=34, bit_width_o=37, binary_point_o=34, latency=0, overflow=Wrap, quantization=Truncate}
      mask prompts: bit_width_i "Bit Width In"; binary_point_i "Binary Point In"; bit_width_o "Bit Width Out"; binary_point_o "Binary Point Out"; overflow "Overflow Behaviour"; quantization "Quantization Behaviour"
      mask help:
      | Converts from one 2's complement bit-width
      | and/or binary point position to another.
      | Includes underflow/overflow indicator.
      mask init: same as c960x4096_x14_7_r2013b_frb/cross_corr/cross_multiplier/cvrt0_0_0_imag
      settings: AttributesFormatString=[37,34]->[37,34]
      mask TypeOptions overflow: Wrap | Saturate | Error
      mask TypeOptions quantization: Truncate | Round  (unbiased: +/- Inf) | Round  (unbiased: even values)
  cvrt1_0_3_real : Subsystem  AncestorBlock=casper_library_misc/convert_of  mask(convert_of){bit_width_i=37, binary_point_i=34, bit_width_o=37, binary_point_o=34, latency=0, overflow=Wrap, quantization=Truncate}
      mask prompts: bit_width_i "Bit Width In"; binary_point_i "Binary Point In"; bit_width_o "Bit Width Out"; binary_point_o "Binary Point Out"; overflow "Overflow Behaviour"; quantization "Quantization Behaviour"
      mask help:
      | Converts from one 2's complement bit-width
      | and/or binary point position to another.
      | Includes underflow/overflow indicator.
      mask init: same as c960x4096_x14_7_r2013b_frb/cross_corr/cross_multiplier/cvrt0_0_0_imag
      settings: AttributesFormatString=[37,34]->[37,34]
      mask TypeOptions overflow: Wrap | Saturate | Error
      mask TypeOptions quantization: Truncate | Round  (unbiased: +/- Inf) | Round  (unbiased: even values)
  cvrt1_0_4_imag : Subsystem  AncestorBlock=casper_library_misc/convert_of  mask(convert_of){bit_width_i=37, binary_point_i=34, bit_width_o=37, binary_point_o=34, latency=0, overflow=Wrap, quantization=Truncate}
      mask prompts: bit_width_i "Bit Width In"; binary_point_i "Binary Point In"; bit_width_o "Bit Width Out"; binary_point_o "Binary Point Out"; overflow "Overflow Behaviour"; quantization "Quantization Behaviour"
      mask help:
      | Converts from one 2's complement bit-width
      | and/or binary point position to another.
      | Includes underflow/overflow indicator.
      mask init: same as c960x4096_x14_7_r2013b_frb/cross_corr/cross_multiplier/cvrt0_0_0_imag
      settings: AttributesFormatString=[37,34]->[37,34]
      mask TypeOptions overflow: Wrap | Saturate | Error
      mask TypeOptions quantization: Truncate | Round  (unbiased: +/- Inf) | Round  (unbiased: even values)
  cvrt1_0_4_real : Subsystem  AncestorBlock=casper_library_misc/convert_of  mask(convert_of){bit_width_i=37, binary_point_i=34, bit_width_o=37, binary_point_o=34, latency=0, overflow=Wrap, quantization=Truncate}
      mask prompts: bit_width_i "Bit Width In"; binary_point_i "Binary Point In"; bit_width_o "Bit Width Out"; binary_point_o "Binary Point Out"; overflow "Overflow Behaviour"; quantization "Quantization Behaviour"
      mask help:
      | Converts from one 2's complement bit-width
      | and/or binary point position to another.
      | Includes underflow/overflow indicator.
      mask init: same as c960x4096_x14_7_r2013b_frb/cross_corr/cross_multiplier/cvrt0_0_0_imag
      settings: AttributesFormatString=[37,34]->[37,34]
      mask TypeOptions overflow: Wrap | Saturate | Error
      mask TypeOptions quantization: Truncate | Round  (unbiased: +/- Inf) | Round  (unbiased: even values)
  cvrt1_0_5_imag : Subsystem  AncestorBlock=casper_library_misc/convert_of  mask(convert_of){bit_width_i=37, binary_point_i=34, bit_width_o=37, binary_point_o=34, latency=0, overflow=Wrap, quantization=Truncate}
      mask prompts: bit_width_i "Bit Width In"; binary_point_i "Binary Point In"; bit_width_o "Bit Width Out"; binary_point_o "Binary Point Out"; overflow "Overflow Behaviour"; quantization "Quantization Behaviour"
      mask help:
      | Converts from one 2's complement bit-width
      | and/or binary point position to another.
      | Includes underflow/overflow indicator.
      mask init: same as c960x4096_x14_7_r2013b_frb/cross_corr/cross_multiplier/cvrt0_0_0_imag
      settings: AttributesFormatString=[37,34]->[37,34]
      mask TypeOptions overflow: Wrap | Saturate | Error
      mask TypeOptions quantization: Truncate | Round  (unbiased: +/- Inf) | Round  (unbiased: even values)
  cvrt1_0_5_real : Subsystem  AncestorBlock=casper_library_misc/convert_of  mask(convert_of){bit_width_i=37, binary_point_i=34, bit_width_o=37, binary_point_o=34, latency=0, overflow=Wrap, quantization=Truncate}
      mask prompts: bit_width_i "Bit Width In"; binary_point_i "Binary Point In"; bit_width_o "Bit Width Out"; binary_point_o "Binary Point Out"; overflow "Overflow Behaviour"; quantization "Quantization Behaviour"
      mask help:
      | Converts from one 2's complement bit-width
      | and/or binary point position to another.
      | Includes underflow/overflow indicator.
      mask init: same as c960x4096_x14_7_r2013b_frb/cross_corr/cross_multiplier/cvrt0_0_0_imag
      settings: AttributesFormatString=[37,34]->[37,34]
      mask TypeOptions overflow: Wrap | Saturate | Error
      mask TypeOptions quantization: Truncate | Round  (unbiased: +/- Inf) | Round  (unbiased: even values)
  cvrt1_0_6_imag : Subsystem  AncestorBlock=casper_library_misc/convert_of  mask(convert_of){bit_width_i=37, binary_point_i=34, bit_width_o=37, binary_point_o=34, latency=0, overflow=Wrap, quantization=Truncate}
      mask prompts: bit_width_i "Bit Width In"; binary_point_i "Binary Point In"; bit_width_o "Bit Width Out"; binary_point_o "Binary Point Out"; overflow "Overflow Behaviour"; quantization "Quantization Behaviour"
      mask help:
      | Converts from one 2's complement bit-width
      | and/or binary point position to another.
      | Includes underflow/overflow indicator.
      mask init: same as c960x4096_x14_7_r2013b_frb/cross_corr/cross_multiplier/cvrt0_0_0_imag
      settings: AttributesFormatString=[37,34]->[37,34]
      mask TypeOptions overflow: Wrap | Saturate | Error
      mask TypeOptions quantization: Truncate | Round  (unbiased: +/- Inf) | Round  (unbiased: even values)
  cvrt1_0_6_real : Subsystem  AncestorBlock=casper_library_misc/convert_of  mask(convert_of){bit_width_i=37, binary_point_i=34, bit_width_o=37, binary_point_o=34, latency=0, overflow=Wrap, quantization=Truncate}
      mask prompts: bit_width_i "Bit Width In"; binary_point_i "Binary Point In"; bit_width_o "Bit Width Out"; binary_point_o "Binary Point Out"; overflow "Overflow Behaviour"; quantization "Quantization Behaviour"
      mask help:
      | Converts from one 2's complement bit-width
      | and/or binary point position to another.
      | Includes underflow/overflow indicator.
      mask init: same as c960x4096_x14_7_r2013b_frb/cross_corr/cross_multiplier/cvrt0_0_0_imag
      settings: AttributesFormatString=[37,34]->[37,34]
      mask TypeOptions overflow: Wrap | Saturate | Error
      mask TypeOptions quantization: Truncate | Round  (unbiased: +/- Inf) | Round  (unbiased: even values)
  cvrt1_0_7_imag : Subsystem  AncestorBlock=casper_library_misc/convert_of  mask(convert_of){bit_width_i=37, binary_point_i=34, bit_width_o=37, binary_point_o=34, latency=0, overflow=Wrap, quantization=Truncate}
      mask prompts: bit_width_i "Bit Width In"; binary_point_i "Binary Point In"; bit_width_o "Bit Width Out"; binary_point_o "Binary Point Out"; overflow "Overflow Behaviour"; quantization "Quantization Behaviour"
      mask help:
      | Converts from one 2's complement bit-width
      | and/or binary point position to another.
      | Includes underflow/overflow indicator.
      mask init: same as c960x4096_x14_7_r2013b_frb/cross_corr/cross_multiplier/cvrt0_0_0_imag
      settings: AttributesFormatString=[37,34]->[37,34]
      mask TypeOptions overflow: Wrap | Saturate | Error
      mask TypeOptions quantization: Truncate | Round  (unbiased: +/- Inf) | Round  (unbiased: even values)
  cvrt1_0_7_real : Subsystem  AncestorBlock=casper_library_misc/convert_of  mask(convert_of){bit_width_i=37, binary_point_i=34, bit_width_o=37, binary_point_o=34, latency=0, overflow=Wrap, quantization=Truncate}
      mask prompts: bit_width_i "Bit Width In"; binary_point_i "Binary Point In"; bit_width_o "Bit Width Out"; binary_point_o "Binary Point Out"; overflow "Overflow Behaviour"; quantization "Quantization Behaviour"
      mask help:
      | Converts from one 2's complement bit-width
      | and/or binary point position to another.
      | Includes underflow/overflow indicator.
      mask init: same as c960x4096_x14_7_r2013b_frb/cross_corr/cross_multiplier/cvrt0_0_0_imag
      settings: AttributesFormatString=[37,34]->[37,34]
      mask TypeOptions overflow: Wrap | Saturate | Error
      mask TypeOptions quantization: Truncate | Round  (unbiased: +/- Inf) | Round  (unbiased: even values)
  delay0_0_0_{0..3} (4 alike) : xbsIndex_r4/Delay  rst=off  infoeditControl=Selection of Reset will increase slice count due to use of real FFs and instead of SRLs  en=off  latency=1  dbl_ovrd=off  reg_retiming=on  block_type=delay
  delay0_0_1_{0..3} (4 alike) : xbsIndex_r4/Delay  rst=off  infoeditControl=Selection of Reset will increase slice count due to use of real FFs and instead of SRLs  en=off  latency=1  dbl_ovrd=off  reg_retiming=on  block_type=delay
  delay0_0_2_{0..3} (4 alike) : xbsIndex_r4/Delay  rst=off  infoeditControl=Selection of Reset will increase slice count due to use of real FFs and instead of SRLs  en=off  latency=1  dbl_ovrd=off  reg_retiming=off  block_type=delay
  delay0_0_3_{0..3} (4 alike) : xbsIndex_r4/Delay  rst=off  infoeditControl=Selection of Reset will increase slice count due to use of real FFs and instead of SRLs  en=off  latency=1  dbl_ovrd=off  reg_retiming=off  block_type=delay
  delay0_0_4_{0..3} (4 alike) : xbsIndex_r4/Delay  rst=off  infoeditControl=Selection of Reset will increase slice count due to use of real FFs and instead of SRLs  en=off  latency=1  dbl_ovrd=off  reg_retiming=off  block_type=delay
  delay0_0_5_{0..3} (4 alike) : xbsIndex_r4/Delay  rst=off  infoeditControl=Selection of Reset will increase slice count due to use of real FFs and instead of SRLs  en=off  latency=1  dbl_ovrd=off  reg_retiming=off  block_type=delay
  delay0_0_6_{0..3} (4 alike) : xbsIndex_r4/Delay  rst=off  infoeditControl=Selection of Reset will increase slice count due to use of real FFs and instead of SRLs  en=off  latency=1  dbl_ovrd=off  reg_retiming=off  block_type=delay
  delay0_0_7_{0..3} (4 alike) : xbsIndex_r4/Delay  rst=off  infoeditControl=Selection of Reset will increase slice count due to use of real FFs and instead of SRLs  en=off  latency=1  dbl_ovrd=off  reg_retiming=off  block_type=delay
  delay0_1_0_{0..3} (4 alike) : xbsIndex_r4/Delay  rst=off  infoeditControl=Selection of Reset will increase slice count due to use of real FFs and instead of SRLs  en=off  latency=1  dbl_ovrd=off  reg_retiming=off  block_type=delay
  delay0_1_1_{0..3} (4 alike) : xbsIndex_r4/Delay  rst=off  infoeditControl=Selection of Reset will increase slice count due to use of real FFs and instead of SRLs  en=off  latency=1  dbl_ovrd=off  reg_retiming=off  block_type=delay
  delay0_1_2_{0..3} (4 alike) : xbsIndex_r4/Delay  rst=off  infoeditControl=Selection of Reset will increase slice count due to use of real FFs and instead of SRLs  en=off  latency=1  dbl_ovrd=off  reg_retiming=off  block_type=delay
  delay0_1_3_{0..3} (4 alike) : xbsIndex_r4/Delay  rst=off  infoeditControl=Selection of Reset will increase slice count due to use of real FFs and instead of SRLs  en=off  latency=1  dbl_ovrd=off  reg_retiming=off  block_type=delay
  delay0_1_4_{0..3} (4 alike) : xbsIndex_r4/Delay  rst=off  infoeditControl=Selection of Reset will increase slice count due to use of real FFs and instead of SRLs  en=off  latency=1  dbl_ovrd=off  reg_retiming=off  block_type=delay
  delay0_1_5_{0..3} (4 alike) : xbsIndex_r4/Delay  rst=off  infoeditControl=Selection of Reset will increase slice count due to use of real FFs and instead of SRLs  en=off  latency=1  dbl_ovrd=off  reg_retiming=off  block_type=delay
  delay0_1_6_{0..3} (4 alike) : xbsIndex_r4/Delay  rst=off  infoeditControl=Selection of Reset will increase slice count due to use of real FFs and instead of SRLs  en=off  latency=1  dbl_ovrd=off  reg_retiming=off  block_type=delay
  delay0_1_7_{0..3} (4 alike) : xbsIndex_r4/Delay  rst=off  infoeditControl=Selection of Reset will increase slice count due to use of real FFs and instead of SRLs  en=off  latency=1  dbl_ovrd=off  reg_retiming=off  block_type=delay
  delay1_0_0_{0..3} (4 alike) : xbsIndex_r4/Delay  rst=off  infoeditControl=Selection of Reset will increase slice count due to use of real FFs and instead of SRLs  en=off  latency=1  dbl_ovrd=off  reg_retiming=on  block_type=delay
  delay1_0_1_{0..3} (4 alike) : xbsIndex_r4/Delay  rst=off  infoeditControl=Selection of Reset will increase slice count due to use of real FFs and instead of SRLs  en=off  latency=1  dbl_ovrd=off  reg_retiming=on  block_type=delay
  delay1_0_2_{0..3} (4 alike) : xbsIndex_r4/Delay  rst=off  infoeditControl=Selection of Reset will increase slice count due to use of real FFs and instead of SRLs  en=off  latency=1  dbl_ovrd=off  reg_retiming=off  block_type=delay
  delay1_0_3_{0..3} (4 alike) : xbsIndex_r4/Delay  rst=off  infoeditControl=Selection of Reset will increase slice count due to use of real FFs and instead of SRLs  en=off  latency=1  dbl_ovrd=off  reg_retiming=off  block_type=delay
  delay1_0_4_{0..3} (4 alike) : xbsIndex_r4/Delay  rst=off  infoeditControl=Selection of Reset will increase slice count due to use of real FFs and instead of SRLs  en=off  latency=1  dbl_ovrd=off  reg_retiming=off  block_type=delay
  delay1_0_5_{0..3} (4 alike) : xbsIndex_r4/Delay  rst=off  infoeditControl=Selection of Reset will increase slice count due to use of real FFs and instead of SRLs  en=off  latency=1  dbl_ovrd=off  reg_retiming=off  block_type=delay
  delay1_0_6_{0..3} (4 alike) : xbsIndex_r4/Delay  rst=off  infoeditControl=Selection of Reset will increase slice count due to use of real FFs and instead of SRLs  en=off  latency=1  dbl_ovrd=off  reg_retiming=off  block_type=delay
  delay1_0_7_{0..3} (4 alike) : xbsIndex_r4/Delay  rst=off  infoeditControl=Selection of Reset will increase slice count due to use of real FFs and instead of SRLs  en=off  latency=1  dbl_ovrd=off  reg_retiming=off  block_type=delay
  pack0_0 : Subsystem  AncestorBlock=casper_library_flow_control/bus_create  mask(bus_create){inputNum=aggregation}
      mask prompts: inputNum "Number of inputs:"
      mask init:
      | bus_create_init(gcb,...
      |     'inputNum', inputNum);
  pack0_1 : Subsystem  AncestorBlock=casper_library_flow_control/bus_create  mask(bus_create){inputNum=aggregation}
      mask prompts: inputNum "Number of inputs:"
      mask init:
      | bus_create_init(gcb,...
      |     'inputNum', inputNum);
  pack1_0 : Subsystem  AncestorBlock=casper_library_flow_control/bus_create  mask(bus_create){inputNum=aggregation}
      mask prompts: inputNum "Number of inputs:"
      mask init:
      | bus_create_init(gcb,...
      |     'inputNum', inputNum);
  ri_to_c0_0_{0..7} (8 alike) : casper_library_misc/ri_to_c
  ri_to_c0_1_{0..7} (8 alike) : casper_library_misc/ri_to_c
  ri_to_c1_0_{0..7} (8 alike) : casper_library_misc/ri_to_c
  sync_delay : xbsIndex_r4/Delay  rst=off  infoeditControl=Selection of Reset will increase slice count due to use of real FFs and instead of SRLs  en=off  latency=mult_latency+add_latency+1+conv_latency  dbl_ovrd=off  reg_retiming=on  block_type=delay
  unpack0 : Subsystem  AncestorBlock=casper_library_flow_control/bus_expand  mask(bus_expand){mode=divisions of equal size, outputNum=aggregation, outputWidth=bit_width_in*2, outputBinaryPt=0, outputArithmeticType=0, show_format=off, outputToWorkspace=off, variablePrefix=out, outputToModelAsWell=on}
      mask prompts: outputNum "Number of outputs:"; outputWidth "Output width:"; outputBinaryPt "Output binary point position:"; outputArithmeticType "Output arithmetic type (ufix=0, fix=1, bool=2):"; show_format "Print format string?"; outputToWorkspace "Output to workspace?"; variablePrefix "Variable name prefix:"; outputToModelAsWell "Output to model as well?"
      mask help:
      | Expands a 'bus' made using a bus_create or Xilinx
      | concat block.
      | The input will be divided into the specified number
      | of outputs with the specified arithmetic types.
      | Divisions are made from most significant bit.
      mask init: same as c960x4096_x14_7_r2013b_frb/ssg/bus_expand
      settings: AttributesFormatString=8 outputs
      mask TypeOptions mode: divisions of equal size | divisions of arbitrary size
      mask Callback mode: bus_expand_callback();
      mask Callback outputWidth: bus_expand_callback();
      mask Callback outputToWorkspace: bus_expand_callback();
  unpack1 : Subsystem  AncestorBlock=casper_library_flow_control/bus_expand  mask(bus_expand){mode=divisions of equal size, outputNum=aggregation, outputWidth=bit_width_in*2, outputBinaryPt=0, outputArithmeticType=0, show_format=off, outputToWorkspace=off, variablePrefix=out, outputToModelAsWell=on}
      mask prompts: outputNum "Number of outputs:"; outputWidth "Output width:"; outputBinaryPt "Output binary point position:"; outputArithmeticType "Output arithmetic type (ufix=0, fix=1, bool=2):"; show_format "Print format string?"; outputToWorkspace "Output to workspace?"; variablePrefix "Variable name prefix:"; outputToModelAsWell "Output to model as well?"
      mask help:
      | Expands a 'bus' made using a bus_create or Xilinx
      | concat block.
      | The input will be divided into the specified number
      | of outputs with the specified arithmetic types.
      | Divisions are made from most significant bit.
      mask init: same as c960x4096_x14_7_r2013b_frb/ssg/bus_expand
      settings: AttributesFormatString=8 outputs
      mask TypeOptions mode: divisions of equal size | divisions of arbitrary size
      mask Callback mode: bus_expand_callback();
      mask Callback outputWidth: bus_expand_callback();
      mask Callback outputToWorkspace: bus_expand_callback();
  sync_out : Outport
  din0_x_din0* : Outport  Port=2
  din0_x_din1* : Outport  Port=3
  din1_x_din1* : Outport  Port=4
  wires:
  sync_in/1 -> sync_delay/1
  sync_delay/1 -> sync_out/1
  din0/1 -> unpack0/1(bus_in)
  unpack0/1(msb_out8) -> c_to_ri0_0/1
  unpack0/2(out7) -> c_to_ri0_1/1
  unpack0/3(out6) -> c_to_ri0_2/1
  unpack0/4(out5) -> c_to_ri0_3/1
  unpack0/5(out4) -> c_to_ri0_4/1
  unpack0/6(out3) -> c_to_ri0_5/1
  unpack0/7(out2) -> c_to_ri0_6/1
  unpack0/8(lsb_out1) -> c_to_ri0_7/1
  din1/1 -> unpack1/1(bus_in)
  unpack1/1(msb_out8) -> c_to_ri1_0/1
  unpack1/2(out7) -> c_to_ri1_1/1
  unpack1/3(out6) -> c_to_ri1_2/1
  unpack1/4(out5) -> c_to_ri1_3/1
  unpack1/5(out4) -> c_to_ri1_4/1
  unpack1/6(out3) -> c_to_ri1_5/1
  unpack1/7(out2) -> c_to_ri1_6/1
  unpack1/8(lsb_out1) -> c_to_ri1_7/1
  c_to_ri0_0/1 -> delay0_0_0_0/1, delay0_0_0_2/1, delay0_1_0_0/1
  delay0_0_0_0/1 -> cmult0_0_0/1
  c_to_ri0_0/2 -> delay0_0_0_1/1, delay0_0_0_3/1, delay0_1_0_1/1
  delay0_0_0_1/1 -> cmult0_0_0/2
  delay0_0_0_2/1 -> cmult0_0_0/3
  delay0_0_0_3/1 -> cmult0_0_0/4
  cmult0_0_0/1 -> cvrt0_0_0_real/1(din)
  cmult0_0_0/2 -> cvrt0_0_0_imag/1(din)
  cvrt0_0_0_real/1(dout) -> ri_to_c0_0_0/1
  cvrt0_0_0_imag/1(dout) -> ri_to_c0_0_0/2
  ri_to_c0_0_0/1 -> pack0_0/1(in1)
  c_to_ri0_1/1 -> delay0_0_1_0/1, delay0_0_1_2/1, delay0_1_1_0/1
  delay0_0_1_0/1 -> cmult0_0_1/1
  c_to_ri0_1/2 -> delay0_0_1_1/1, delay0_0_1_3/1, delay0_1_1_1/1
  delay0_0_1_1/1 -> cmult0_0_1/2
  delay0_0_1_2/1 -> cmult0_0_1/3
  delay0_0_1_3/1 -> cmult0_0_1/4
  cmult0_0_1/1 -> cvrt0_0_1_real/1(din)
  cmult0_0_1/2 -> cvrt0_0_1_imag/1(din)
  cvrt0_0_1_real/1(dout) -> ri_to_c0_0_1/1
  cvrt0_0_1_imag/1(dout) -> ri_to_c0_0_1/2
  ri_to_c0_0_1/1 -> pack0_0/2(in2)
  c_to_ri0_2/1 -> delay0_0_2_0/1, delay0_0_2_2/1, delay0_1_2_0/1
  delay0_0_2_0/1 -> cmult0_0_2/1
  c_to_ri0_2/2 -> delay0_0_2_1/1, delay0_0_2_3/1, delay0_1_2_1/1
  delay0_0_2_1/1 -> cmult0_0_2/2
  delay0_0_2_2/1 -> cmult0_0_2/3
  delay0_0_2_3/1 -> cmult0_0_2/4
  cmult0_0_2/1 -> cvrt0_0_2_real/1(din)
  cmult0_0_2/2 -> cvrt0_0_2_imag/1(din)
  cvrt0_0_2_real/1(dout) -> ri_to_c0_0_2/1
  cvrt0_0_2_imag/1(dout) -> ri_to_c0_0_2/2
  ri_to_c0_0_2/1 -> pack0_0/3(in3)
  c_to_ri0_3/1 -> delay0_0_3_0/1, delay0_0_3_2/1, delay0_1_3_0/1
  delay0_0_3_0/1 -> cmult0_0_3/1
  c_to_ri0_3/2 -> delay0_0_3_1/1, delay0_0_3_3/1, delay0_1_3_1/1
  delay0_0_3_1/1 -> cmult0_0_3/2
  delay0_0_3_2/1 -> cmult0_0_3/3
  delay0_0_3_3/1 -> cmult0_0_3/4
  cmult0_0_3/1 -> cvrt0_0_3_real/1(din)
  cmult0_0_3/2 -> cvrt0_0_3_imag/1(din)
  cvrt0_0_3_real/1(dout) -> ri_to_c0_0_3/1
  cvrt0_0_3_imag/1(dout) -> ri_to_c0_0_3/2
  ri_to_c0_0_3/1 -> pack0_0/4(in4)
  c_to_ri0_4/1 -> delay0_0_4_0/1, delay0_0_4_2/1, delay0_1_4_0/1
  delay0_0_4_0/1 -> cmult0_0_4/1
  c_to_ri0_4/2 -> delay0_0_4_1/1, delay0_0_4_3/1, delay0_1_4_1/1
  delay0_0_4_1/1 -> cmult0_0_4/2
  delay0_0_4_2/1 -> cmult0_0_4/3
  delay0_0_4_3/1 -> cmult0_0_4/4
  cmult0_0_4/1 -> cvrt0_0_4_real/1(din)
  cmult0_0_4/2 -> cvrt0_0_4_imag/1(din)
  cvrt0_0_4_real/1(dout) -> ri_to_c0_0_4/1
  cvrt0_0_4_imag/1(dout) -> ri_to_c0_0_4/2
  ri_to_c0_0_4/1 -> pack0_0/5(in5)
  c_to_ri0_5/1 -> delay0_0_5_0/1, delay0_0_5_2/1, delay0_1_5_0/1
  delay0_0_5_0/1 -> cmult0_0_5/1
  c_to_ri0_5/2 -> delay0_0_5_1/1, delay0_0_5_3/1, delay0_1_5_1/1
  delay0_0_5_1/1 -> cmult0_0_5/2
  delay0_0_5_2/1 -> cmult0_0_5/3
  delay0_0_5_3/1 -> cmult0_0_5/4
  cmult0_0_5/1 -> cvrt0_0_5_real/1(din)
  cmult0_0_5/2 -> cvrt0_0_5_imag/1(din)
  cvrt0_0_5_real/1(dout) -> ri_to_c0_0_5/1
  cvrt0_0_5_imag/1(dout) -> ri_to_c0_0_5/2
  ri_to_c0_0_5/1 -> pack0_0/6(in6)
  c_to_ri0_6/1 -> delay0_0_6_0/1, delay0_0_6_2/1, delay0_1_6_0/1
  delay0_0_6_0/1 -> cmult0_0_6/1
  c_to_ri0_6/2 -> delay0_0_6_1/1, delay0_0_6_3/1, delay0_1_6_1/1
  delay0_0_6_1/1 -> cmult0_0_6/2
  delay0_0_6_2/1 -> cmult0_0_6/3
  delay0_0_6_3/1 -> cmult0_0_6/4
  cmult0_0_6/1 -> cvrt0_0_6_real/1(din)
  cmult0_0_6/2 -> cvrt0_0_6_imag/1(din)
  cvrt0_0_6_real/1(dout) -> ri_to_c0_0_6/1
  cvrt0_0_6_imag/1(dout) -> ri_to_c0_0_6/2
  ri_to_c0_0_6/1 -> pack0_0/7(in7)
  c_to_ri0_7/1 -> delay0_0_7_0/1, delay0_0_7_2/1, delay0_1_7_0/1
  delay0_0_7_0/1 -> cmult0_0_7/1
  c_to_ri0_7/2 -> delay0_0_7_1/1, delay0_0_7_3/1, delay0_1_7_1/1
  delay0_0_7_1/1 -> cmult0_0_7/2
  delay0_0_7_2/1 -> cmult0_0_7/3
  delay0_0_7_3/1 -> cmult0_0_7/4
  cmult0_0_7/1 -> cvrt0_0_7_real/1(din)
  cmult0_0_7/2 -> cvrt0_0_7_imag/1(din)
  cvrt0_0_7_real/1(dout) -> ri_to_c0_0_7/1
  cvrt0_0_7_imag/1(dout) -> ri_to_c0_0_7/2
  ri_to_c0_0_7/1 -> pack0_0/8(in8)
  pack0_0/1(bus_out) -> din0_x_din0*/1
  delay0_1_0_0/1 -> cmult0_1_0/1
  delay0_1_0_1/1 -> cmult0_1_0/2
  c_to_ri1_0/1 -> delay0_1_0_2/1, delay1_0_0_0/1, delay1_0_0_2/1
  delay0_1_0_2/1 -> cmult0_1_0/3
  c_to_ri1_0/2 -> delay0_1_0_3/1, delay1_0_0_1/1, delay1_0_0_3/1
  delay0_1_0_3/1 -> cmult0_1_0/4
  cmult0_1_0/1 -> cvrt0_1_0_real/1(din)
  cmult0_1_0/2 -> cvrt0_1_0_imag/1(din)
  cvrt0_1_0_real/1(dout) -> ri_to_c0_1_0/1
  cvrt0_1_0_imag/1(dout) -> ri_to_c0_1_0/2
  ri_to_c0_1_0/1 -> pack0_1/1(in1)
  delay0_1_1_0/1 -> cmult0_1_1/1
  delay0_1_1_1/1 -> cmult0_1_1/2
  c_to_ri1_1/1 -> delay0_1_1_2/1, delay1_0_1_0/1, delay1_0_1_2/1
  delay0_1_1_2/1 -> cmult0_1_1/3
  c_to_ri1_1/2 -> delay0_1_1_3/1, delay1_0_1_1/1, delay1_0_1_3/1
  delay0_1_1_3/1 -> cmult0_1_1/4
  cmult0_1_1/1 -> cvrt0_1_1_real/1(din)
  cmult0_1_1/2 -> cvrt0_1_1_imag/1(din)
  cvrt0_1_1_real/1(dout) -> ri_to_c0_1_1/1
  cvrt0_1_1_imag/1(dout) -> ri_to_c0_1_1/2
  ri_to_c0_1_1/1 -> pack0_1/2(in2)
  delay0_1_2_0/1 -> cmult0_1_2/1
  delay0_1_2_1/1 -> cmult0_1_2/2
  c_to_ri1_2/1 -> delay0_1_2_2/1, delay1_0_2_0/1, delay1_0_2_2/1
  delay0_1_2_2/1 -> cmult0_1_2/3
  c_to_ri1_2/2 -> delay0_1_2_3/1, delay1_0_2_1/1, delay1_0_2_3/1
  delay0_1_2_3/1 -> cmult0_1_2/4
  cmult0_1_2/1 -> cvrt0_1_2_real/1(din)
  cmult0_1_2/2 -> cvrt0_1_2_imag/1(din)
  cvrt0_1_2_real/1(dout) -> ri_to_c0_1_2/1
  cvrt0_1_2_imag/1(dout) -> ri_to_c0_1_2/2
  ri_to_c0_1_2/1 -> pack0_1/3(in3)
  delay0_1_3_0/1 -> cmult0_1_3/1
  delay0_1_3_1/1 -> cmult0_1_3/2
  c_to_ri1_3/1 -> delay0_1_3_2/1, delay1_0_3_0/1, delay1_0_3_2/1
  delay0_1_3_2/1 -> cmult0_1_3/3
  c_to_ri1_3/2 -> delay0_1_3_3/1, delay1_0_3_1/1, delay1_0_3_3/1
  delay0_1_3_3/1 -> cmult0_1_3/4
  cmult0_1_3/1 -> cvrt0_1_3_real/1(din)
  cmult0_1_3/2 -> cvrt0_1_3_imag/1(din)
  cvrt0_1_3_real/1(dout) -> ri_to_c0_1_3/1
  cvrt0_1_3_imag/1(dout) -> ri_to_c0_1_3/2
  ri_to_c0_1_3/1 -> pack0_1/4(in4)
  delay0_1_4_0/1 -> cmult0_1_4/1
  delay0_1_4_1/1 -> cmult0_1_4/2
  c_to_ri1_4/1 -> delay0_1_4_2/1, delay1_0_4_0/1, delay1_0_4_2/1
  delay0_1_4_2/1 -> cmult0_1_4/3
  c_to_ri1_4/2 -> delay0_1_4_3/1, delay1_0_4_1/1, delay1_0_4_3/1
  delay0_1_4_3/1 -> cmult0_1_4/4
  cmult0_1_4/1 -> cvrt0_1_4_real/1(din)
  cmult0_1_4/2 -> cvrt0_1_4_imag/1(din)
  cvrt0_1_4_real/1(dout) -> ri_to_c0_1_4/1
  cvrt0_1_4_imag/1(dout) -> ri_to_c0_1_4/2
  ri_to_c0_1_4/1 -> pack0_1/5(in5)
  delay0_1_5_0/1 -> cmult0_1_5/1
  delay0_1_5_1/1 -> cmult0_1_5/2
  c_to_ri1_5/1 -> delay0_1_5_2/1, delay1_0_5_0/1, delay1_0_5_2/1
  delay0_1_5_2/1 -> cmult0_1_5/3
  c_to_ri1_5/2 -> delay0_1_5_3/1, delay1_0_5_1/1, delay1_0_5_3/1
  delay0_1_5_3/1 -> cmult0_1_5/4
  cmult0_1_5/1 -> cvrt0_1_5_real/1(din)
  cmult0_1_5/2 -> cvrt0_1_5_imag/1(din)
  cvrt0_1_5_real/1(dout) -> ri_to_c0_1_5/1
  cvrt0_1_5_imag/1(dout) -> ri_to_c0_1_5/2
  ri_to_c0_1_5/1 -> pack0_1/6(in6)
  delay0_1_6_0/1 -> cmult0_1_6/1
  delay0_1_6_1/1 -> cmult0_1_6/2
  c_to_ri1_6/1 -> delay0_1_6_2/1, delay1_0_6_0/1, delay1_0_6_2/1
  delay0_1_6_2/1 -> cmult0_1_6/3
  c_to_ri1_6/2 -> delay0_1_6_3/1, delay1_0_6_1/1, delay1_0_6_3/1
  delay0_1_6_3/1 -> cmult0_1_6/4
  cmult0_1_6/1 -> cvrt0_1_6_real/1(din)
  cmult0_1_6/2 -> cvrt0_1_6_imag/1(din)
  cvrt0_1_6_real/1(dout) -> ri_to_c0_1_6/1
  cvrt0_1_6_imag/1(dout) -> ri_to_c0_1_6/2
  ri_to_c0_1_6/1 -> pack0_1/7(in7)
  delay0_1_7_0/1 -> cmult0_1_7/1
  delay0_1_7_1/1 -> cmult0_1_7/2
  c_to_ri1_7/1 -> delay0_1_7_2/1, delay1_0_7_0/1, delay1_0_7_2/1
  delay0_1_7_2/1 -> cmult0_1_7/3
  c_to_ri1_7/2 -> delay0_1_7_3/1, delay1_0_7_1/1, delay1_0_7_3/1
  delay0_1_7_3/1 -> cmult0_1_7/4
  cmult0_1_7/1 -> cvrt0_1_7_real/1(din)
  cmult0_1_7/2 -> cvrt0_1_7_imag/1(din)
  cvrt0_1_7_real/1(dout) -> ri_to_c0_1_7/1
  cvrt0_1_7_imag/1(dout) -> ri_to_c0_1_7/2
  ri_to_c0_1_7/1 -> pack0_1/8(in8)
  pack0_1/1(bus_out) -> din0_x_din1*/1
  delay1_0_0_0/1 -> cmult1_0_0/1
  delay1_0_0_1/1 -> cmult1_0_0/2
  delay1_0_0_2/1 -> cmult1_0_0/3
  delay1_0_0_3/1 -> cmult1_0_0/4
  cmult1_0_0/1 -> cvrt1_0_0_real/1(din)
  cmult1_0_0/2 -> cvrt1_0_0_imag/1(din)
  cvrt1_0_0_real/1(dout) -> ri_to_c1_0_0/1
  cvrt1_0_0_imag/1(dout) -> ri_to_c1_0_0/2
  ri_to_c1_0_0/1 -> pack1_0/1(in1)
  delay1_0_1_0/1 -> cmult1_0_1/1
  delay1_0_1_1/1 -> cmult1_0_1/2
  delay1_0_1_2/1 -> cmult1_0_1/3
  delay1_0_1_3/1 -> cmult1_0_1/4
  cmult1_0_1/1 -> cvrt1_0_1_real/1(din)
  cmult1_0_1/2 -> cvrt1_0_1_imag/1(din)
  cvrt1_0_1_real/1(dout) -> ri_to_c1_0_1/1
  cvrt1_0_1_imag/1(dout) -> ri_to_c1_0_1/2
  ri_to_c1_0_1/1 -> pack1_0/2(in2)
  delay1_0_2_0/1 -> cmult1_0_2/1
  delay1_0_2_1/1 -> cmult1_0_2/2
  delay1_0_2_2/1 -> cmult1_0_2/3
  delay1_0_2_3/1 -> cmult1_0_2/4
  cmult1_0_2/1 -> cvrt1_0_2_real/1(din)
  cmult1_0_2/2 -> cvrt1_0_2_imag/1(din)
  cvrt1_0_2_real/1(dout) -> ri_to_c1_0_2/1
  cvrt1_0_2_imag/1(dout) -> ri_to_c1_0_2/2
  ri_to_c1_0_2/1 -> pack1_0/3(in3)
  delay1_0_3_0/1 -> cmult1_0_3/1
  delay1_0_3_1/1 -> cmult1_0_3/2
  delay1_0_3_2/1 -> cmult1_0_3/3
  delay1_0_3_3/1 -> cmult1_0_3/4
  cmult1_0_3/1 -> cvrt1_0_3_real/1(din)
  cmult1_0_3/2 -> cvrt1_0_3_imag/1(din)
  cvrt1_0_3_real/1(dout) -> ri_to_c1_0_3/1
  cvrt1_0_3_imag/1(dout) -> ri_to_c1_0_3/2
  ri_to_c1_0_3/1 -> pack1_0/4(in4)
  delay1_0_4_0/1 -> cmult1_0_4/1
  delay1_0_4_1/1 -> cmult1_0_4/2
  delay1_0_4_2/1 -> cmult1_0_4/3
  delay1_0_4_3/1 -> cmult1_0_4/4
  cmult1_0_4/1 -> cvrt1_0_4_real/1(din)
  cmult1_0_4/2 -> cvrt1_0_4_imag/1(din)
  cvrt1_0_4_real/1(dout) -> ri_to_c1_0_4/1
  cvrt1_0_4_imag/1(dout) -> ri_to_c1_0_4/2
  ri_to_c1_0_4/1 -> pack1_0/5(in5)
  delay1_0_5_0/1 -> cmult1_0_5/1
  delay1_0_5_1/1 -> cmult1_0_5/2
  delay1_0_5_2/1 -> cmult1_0_5/3
  delay1_0_5_3/1 -> cmult1_0_5/4
  cmult1_0_5/1 -> cvrt1_0_5_real/1(din)
  cmult1_0_5/2 -> cvrt1_0_5_imag/1(din)
  cvrt1_0_5_real/1(dout) -> ri_to_c1_0_5/1
  cvrt1_0_5_imag/1(dout) -> ri_to_c1_0_5/2
  ri_to_c1_0_5/1 -> pack1_0/6(in6)
  delay1_0_6_0/1 -> cmult1_0_6/1
  delay1_0_6_1/1 -> cmult1_0_6/2
  delay1_0_6_2/1 -> cmult1_0_6/3
  delay1_0_6_3/1 -> cmult1_0_6/4
  cmult1_0_6/1 -> cvrt1_0_6_real/1(din)
  cmult1_0_6/2 -> cvrt1_0_6_imag/1(din)
  cvrt1_0_6_real/1(dout) -> ri_to_c1_0_6/1
  cvrt1_0_6_imag/1(dout) -> ri_to_c1_0_6/2
  ri_to_c1_0_6/1 -> pack1_0/7(in7)
  delay1_0_7_0/1 -> cmult1_0_7/1
  delay1_0_7_1/1 -> cmult1_0_7/2
  delay1_0_7_2/1 -> cmult1_0_7/3
  delay1_0_7_3/1 -> cmult1_0_7/4
  cmult1_0_7/1 -> cvrt1_0_7_real/1(din)
  cmult1_0_7/2 -> cvrt1_0_7_imag/1(din)
  cvrt1_0_7_real/1(dout) -> ri_to_c1_0_7/1
  cvrt1_0_7_imag/1(dout) -> ri_to_c1_0_7/2
  ri_to_c1_0_7/1 -> pack1_0/8(in8)
  pack1_0/1(bus_out) -> din1_x_din1*/1
